simulink model "FMrec"  (Simulink 9.0)
settings: Solver=FixedStepDiscrete  StartTime=0.0  StopTime=1000  RelTol=1e-3
PreLoadFcn:
  | setenv('MW_MINGW64_LOC','C:\TDM-GCC-64')
StartFcn:
  | tic
StopFcn:
  | toc;
undefined symbols (not defined in the file): magnitude
libraries: UN_HIL_Lib x2, dsparch4 x2, dspobslib x1
Description:
  | QPSK Transmitter and Receiver.
  | 
  | This model shows the implementation of a QPSK transmitter and receiver.
settings Model: FPTRunName=Active  Creator=The MathWorks Inc.  LastModifiedBy=minel
settings DataIOCC: LimitDataPoints=on  SignalLoggingSaveFormat=ModelDataLogs  SaveOutput=off  SaveTime=off
settings OptimizationCC: BooleanDataType=off  DefaultParameterBehavior=Inlined  ExpressionDepthLimit=2147483647  LocalBlockOutputs=off
settings DebuggingCC: AlgebraicLoopMsg=error  SolverPrmCheckMsg=warning  SingleTaskRateTransMsg=error  ParameterPrecisionLossMsg=none  FcnCallInpInsideContextMsg=warning  StateNameClashWarn=warning
settings HardwareCC: TargetBitPerPointer=64  TargetBitPerSizeT=64  TargetBitPerPtrDiffT=64  TargetLongLongMode=on  TargetIntDivRoundTo=Zero  TargetEndianess=LittleEndian  TargetWordSize=64  TargetHWDeviceType=Generic->MATLAB Host Computer  ProdEqTarget=off
settings GRTTargetCC: GeneratePreprocessorConditionals=Disable all
settings ConfigComp: CovSFcnEnable=off
settings SimEventsCC: propDiagStatOutput=1  propPreventDuplicateEvents=0

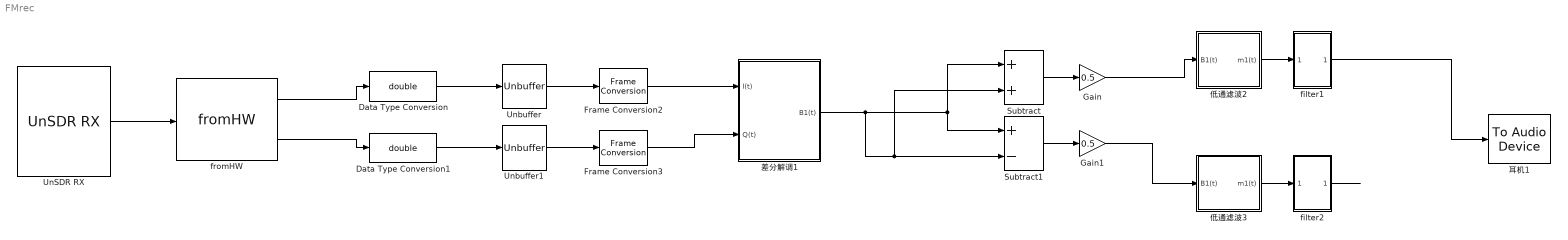
== system FMrec ==
  Data Type Conversion : DataTypeConversion  OutDataTypeStr=double
  Data Type Conversion1 : DataTypeConversion  OutDataTypeStr=double
  Frame Conversion2 : FrameConversion  InheritSamplingMode=off  OutFrame=Sample-based
  Frame Conversion3 : FrameConversion  InheritSamplingMode=off  OutFrame=Sample-based
  Gain : Gain  Gain=0.5
  Gain1 : Gain  Gain=0.5
  Subtract : Sum
  Subtract1 : Sum  Inputs=+-
  UnSDR RX : UN_HIL_Lib/UnSDR RX  SystemSampleTime=-1
      settings: SourceProductName=HIL Blockset
  Unbuffer : Unbuffer
  Unbuffer1 : Unbuffer
  filter1 : Subsystem
  filter2 : Subsystem
  fromHW : UN_HIL_Lib/fromHW  sp=1/144e3
      settings: SourceProductName=HIL Blockset
  低通滤波2 : Subsystem
  低通滤波3 : Subsystem
  差分解调1 : Subsystem
  耳机1 : dspobslib/To Audio Device  deviceName=扬声器/听筒 (Realtek Audio)  inheritSampleRate=on  sampleRate=44100  deviceDatatype=Determine from input data type  autoBufferSize=on  bufferSize=4096  queueDuration=2  defaultOutputChannelMapping=on  outputChannelMapping=1:2  outputNumUnderrunSamples=off
      settings: SourceProductName=DSP System Toolbox  SourceProductBaseCode=DS
  wires:
  Unbuffer/1 -> Frame Conversion2/1
  fromHW/1 -> Data Type Conversion/1
  Data Type Conversion/1 -> Unbuffer/1
  fromHW/2 -> Data Type Conversion1/1
  Data Type Conversion1/1 -> Unbuffer1/1
  Unbuffer1/1 -> Frame Conversion3/1
  UnSDR RX/1 -> fromHW/1
  低通滤波3/1(m1(t)) -> filter2/1(In1)
  filter2/1(Out1) -> ?
  filter1/1(Out1) -> 耳机1/1
  低通滤波2/1(m1(t)) -> filter1/1(In1)
  Frame Conversion2/1 -> 差分解调1/1(I(t))
  Gain/1 -> 低通滤波2/1(B1(t))
  Gain1/1 -> 低通滤波3/1(B1(t))
  Subtract1/1 -> Gain1/1
  Subtract/1 -> Gain/1
  差分解调1/1(B1(t)) -> Subtract/2, Subtract1/2, Subtract/1, Subtract1/1
  Frame Conversion3/1 -> 差分解调1/2(Q(t))

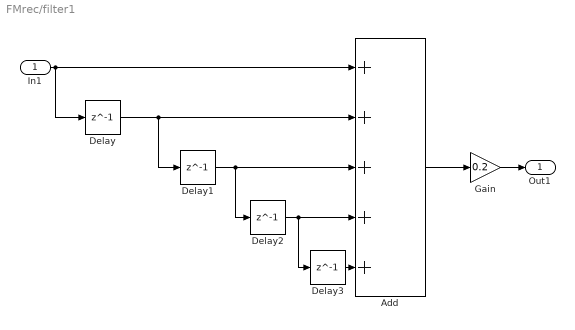
== system FMrec/filter1 ==
  In1 : Inport
  Add : Sum  Inputs=+++++
  Delay{,1..3} (4 alike) : Delay  DelayLength=1  InitialCondition=0
  Gain : Gain  Gain=0.2
  Out1 : Outport
  wires:
  In1/1 -> Add/1, Delay/1
  Add/1 -> Gain/1
  Gain/1 -> Out1/1
  Delay/1 -> Delay1/1, Add/2
  Delay1/1 -> Delay2/1, Add/3
  Delay2/1 -> Delay3/1, Add/4
  Delay3/1 -> Add/5

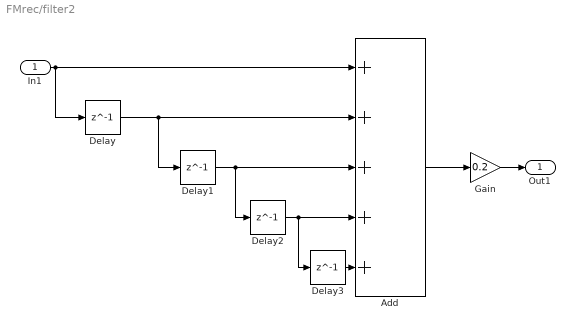
== system FMrec/filter2 ==
  In1 : Inport
  Add : Sum  Inputs=+++++
  Delay{,1..3} (4 alike) : Delay  DelayLength=1  InitialCondition=0
  Gain : Gain  Gain=0.2
  Out1 : Outport
  wires:
  In1/1 -> Add/1, Delay/1
  Add/1 -> Gain/1
  Gain/1 -> Out1/1
  Delay/1 -> Delay1/1, Add/2
  Delay1/1 -> Delay2/1, Add/3
  Delay2/1 -> Delay3/1, Add/4
  Delay3/1 -> Add/5

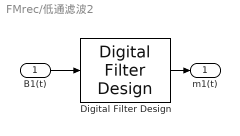
== system FMrec/低通滤波2 ==
  B1(t) : Inport
  Digital Filter Design : dsparch4/Digital Filter Design  mwdsp_browser_bugfix_var=off
  m1(t) : Outport
  wires:
  Digital Filter Design/1 -> m1(t)/1
  B1(t)/1 -> Digital Filter Design/1

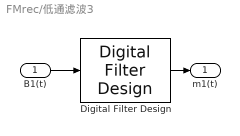
== system FMrec/低通滤波3 ==
  B1(t) : Inport
  Digital Filter Design : dsparch4/Digital Filter Design  mwdsp_browser_bugfix_var=off
  m1(t) : Outport
  wires:
  Digital Filter Design/1 -> m1(t)/1
  B1(t)/1 -> Digital Filter Design/1

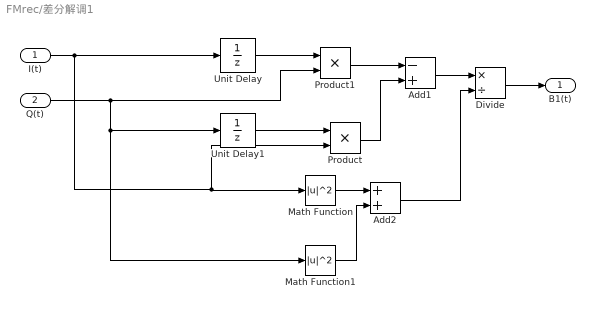
== system FMrec/差分解调1 ==
  I(t) : Inport
  Q(t) : Inport  Port=2
  Add1 : Sum  Inputs=-+
  Add2 : Sum
  Divide : Product  Inputs=*/
  Math Function : Math  Operator=magnitude^2  SaturateOnIntegerOverflow=on
  Math Function1 : Math  Operator=magnitude^2  SaturateOnIntegerOverflow=on
  Product : Product  RndMeth=Zero
  Product1 : Product  RndMeth=Zero
  Unit Delay : UnitDelay  SampleTime=-1
  Unit Delay1 : UnitDelay  SampleTime=-1
  B1(t) : Outport
  wires:
  Add1/1 -> Divide/1
  Add2/1 -> Divide/2
  Product/1 -> Add1/2
  Product1/1 -> Add1/1
  Unit Delay/1 -> Product1/1
  Unit Delay1/1 -> Product/1
  Q(t)/1 -> Math Function1/1, Unit Delay1/1, Product1/2
  I(t)/1 -> Product/2, Math Function/1, Unit Delay/1
  Math Function/1 -> Add2/1
  Math Function1/1 -> Add2/2
  Divide/1 -> B1(t)/1
